simulink model "Gear_Chain"  (R2014a)
settings: Solver=ode45  StartTime=0.0  StopTime=10.0  RelTol=1e-3
model workspace: external: MAT-File Vehicle\Gear_Chain\Data\Gear_Chain.mat (data not in the file)
undefined symbols (not defined in the file): ceffx, ceffy, Jc, Jg, Jm, Jt, Rg, w0
settings Model: Creator=Nathan  LastModifiedBy=Nathan
settings OptimizationCC: InlineParams=on
settings DebuggingCC: UnderspecifiedInitializationDetection=Classic  StateNameClashWarn=warning
settings ModelReferenceCC: ModelReferenceMinAlgLoopOccurrences=on

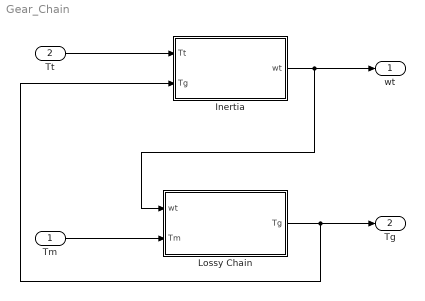
== system Gear_Chain ==
  Tm : Inport
  Tt : Inport  Port=2
  Inertia : Subsystem
  Lossy Chain : Subsystem
  wt : Outport
  Tg : Outport  Port=2
  wires:
  Tm/1 -> Lossy Chain/2(Tm)
  Tt/1 -> Inertia/1(Tt)
  Inertia/1(wt) -> Lossy Chain/1(wt), wt/1
  Lossy Chain/1(Tg) -> Inertia/2(Tg), Tg/1

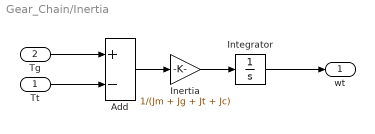
== system Gear_Chain/Inertia ==
  Tt : Inport
  Tg : Inport  Port=2
  Add : Sum  Inputs=+-
  Inertia : Gain  Gain=1/(Jm + Jg + Jt + Jc)
  Integrator : Integrator  InitialCondition=w0
  wt : Outport
  wires:
  Tt/1 -> Add/2
  Tg/1 -> Add/1
  Inertia/1 -> Integrator/1
  Integrator/1 -> wt/1
  Add/1 -> Inertia/1

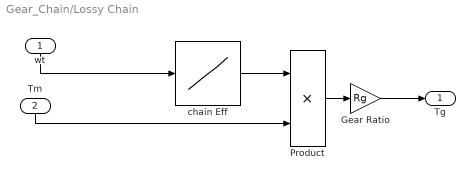
== system Gear_Chain/Lossy Chain ==
  wt : Inport
  Tm : Inport  Port=2
  Gear Ratio : Gain  Gain=Rg
  Product : Product
  chain Eff : Lookup_n-D  NumberOfTableDimensions=1  BreakpointsForDimension1=ceffx  Table=ceffy  RndMeth=Simplest  InputSameDT=on
  Tg : Outport
  wires:
  Tm/1 -> Product/2
  wt/1 -> chain Eff/1
  Product/1 -> Gear Ratio/1
  chain Eff/1 -> Product/1
  Gear Ratio/1 -> Tg/1
